simulink model "UUV_animation"  (Simulink 8.3)
settings: Solver=ode45  StartTime=0.0  StopTime=1000  RelTol=1e-3
undefined symbols (not defined in the file or in its folder): drawUUV
libraries: simulink x1
settings Model: Creator=beard  LastModifiedBy=jhl48
settings OptimizationCC: ExpressionDepthLimit=2147483647  InitFltsAndDblsToZero=on
settings DebuggingCC: FcnCallInpInsideContextMsg=UseLocalSettings

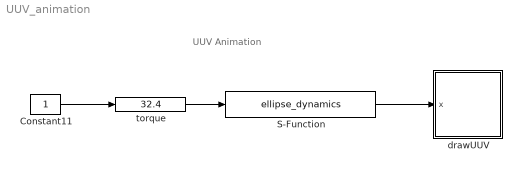
== system UUV_animation ==
  note: UUV Animation
  Constant11 : Constant
  S-Function : S-Function  FunctionName=ellipse_dynamics  Parameters=AP  EnableBusSupport=off
  drawUUV : Subsystem
      mask init:
      | % drawing parameters
      | MajorAxis = 10;
      | MinorAxis = 6;
      | C_M = [0;-4];
      mask Display: image(imread('tv.jpg'))
  torque : simulink/Math Operations/Slider Gain  low=-180  gain=32.4  high=180
  wires:
  Constant11/1 -> torque/1
  torque/1 -> S-Function/1
  S-Function/1 -> drawUUV/1(x)

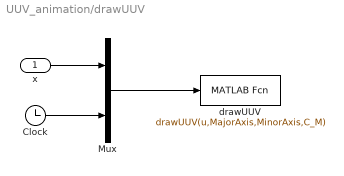
== system UUV_animation/drawUUV ==
  x : Inport
  Clock : Clock
  Mux : Mux  Inputs=2
  drawUUV : MATLABFcn  MATLABFcn=drawUUV(u,MajorAxis,MinorAxis,C_M)  OutputDimensions=0  SampleTime=0.1
  wires:
  Mux/1 -> drawUUV/1
  x/1 -> Mux/1
  Clock/1 -> Mux/2
